simulink model "Pyramidal_Config_Model"  (R2024b)
settings: Solver=VariableStepAuto  StartTime=0.0  StopTime=50  FixedStep=0.001  RelTol=1e-3
libraries: slpidlib x7, simulink_extras x2, aerolibutil x1
settings Model: Creator=LEGION  LastModifiedBy=LEGION

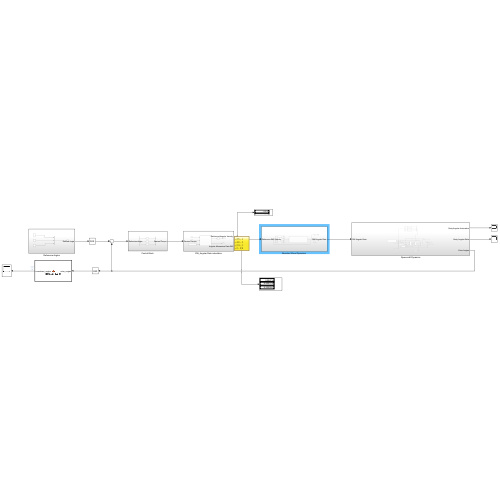
[thumbnail: Simulink's stored preview of the top-level diagram]
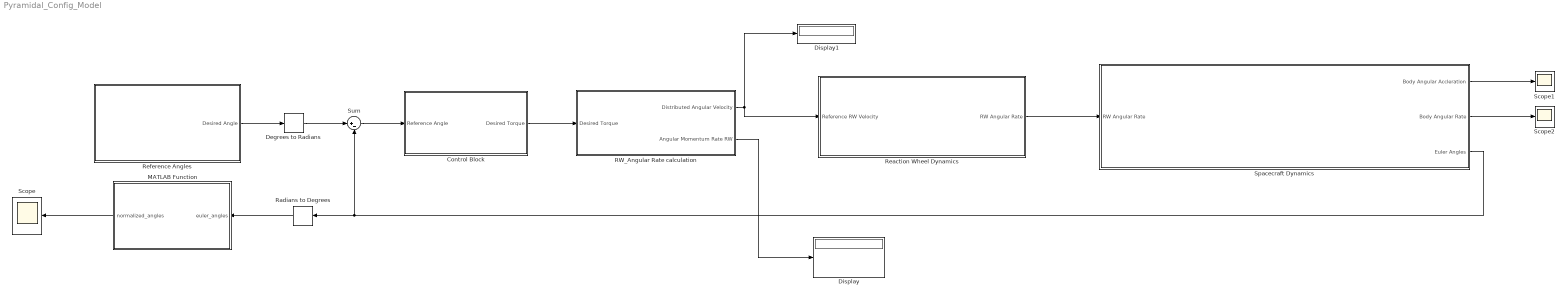
== system Pyramidal_Config_Model ==
  Control Block : Subsystem
  Degrees to Radians : simulink_extras/Transformations/Degrees to Radians
  Display : Display
  Display1 : Display
  MATLAB Function : MATLAB Function  TreatAsAtomicUnit=on
  RW_Angular Rate calculation : Subsystem
  Radians to Degrees : simulink_extras/Transformations/Radians to Degrees
  "Reaction Wheel Dynamics " : Subsystem
  Reference Angles : Subsystem
  Scope : Scope
  Scope1 : Scope
  Scope2 : Scope
  Spacecraft Dynamics : Subsystem
  Sum : Sum  Inputs=|+-
  wires:
  Degrees to Radians/1 -> Sum/1
  Sum/1 -> Control Block/1(Reference Angle)
  Control Block/1(Desired Torque) -> RW_Angular Rate calculation/1(Desired Torque)
  RW_Angular Rate calculation/1(Distributed Angular Velocity) -> Display1/1, "Reaction Wheel Dynamics "/1(Reference RW Velocity)
  MATLAB Function/1(normalized_angles) -> Scope/1
  Spacecraft Dynamics/1(Body Angular Accleration) -> Scope1/1
  Spacecraft Dynamics/2(Body Angular Rate) -> Scope2/1
  RW_Angular Rate calculation/2(Angular Momentum Rate RW) -> Display/1
  Spacecraft Dynamics/3(Euler Angles) -> Sum/2, Radians to Degrees/1
  Radians to Degrees/1 -> MATLAB Function/1(euler_angles)
  Reference Angles/1(Desired Angle) -> Degrees to Radians/1
  "Reaction Wheel Dynamics "/1(RW Angular Rate) -> Spacecraft Dynamics/1(RW Angular Rate)

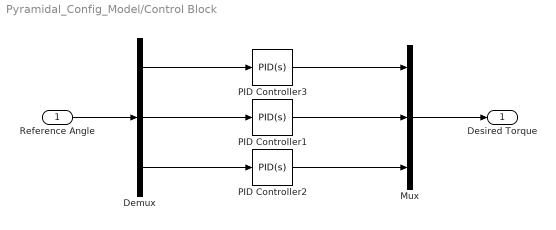
== system Pyramidal_Config_Model/Control Block ==
  Reference Angle : Inport
  Demux : Demux  Outputs=3
  Mux : Mux  Inputs=3
  PID Controller1 : slpidlib/PID Controller  Controller=PID  Form=Parallel  TimeDomain=Continuous-time  UseExternalTs=off  SampleTime=-1  IntegratorMethod=Forward Euler  FilterMethod=Forward Euler  ControllerParametersSource=internal  P=0.1  I=0.05  UseKiTs=off  D=0.01  UseExternalDerivativeSource=off  N=100  UseFilter=on  TunerSelectOption=Transfer Function Based (PID Tuner App)  InitialConditionSource=internal  InitialConditionForIntegrator=0  InitialConditionForFilter=0  DifferentiatorICPrevScaledInput=0  ExternalReset=none  TrackingMode=off  Kt=1  LimitOutput=off  SatLimitsSource=internal  UpperSaturationLimit=inf  LowerSaturationLimit=-inf  LinearizeAsGain=on  AntiWindupMode=none  Kb=1  LimitIntegrator=off  UpperIntegratorSaturationLimit=inf  LowerIntegratorSaturationLimit=-inf  POutMin=[]  POutMax=[]  IOutMin=[]  IOutMax=[]  DOutMin=[]  DOutMax=[]  NOutMin=[]  NOutMax=[]  SumOutMin=[]  SumOutMax=[]  SaturationOutMin=[]  SaturationOutMax=[]  PParamMin=[]  PParamMax=[]  IParamMin=[]  IParamMax=[]  DParamMin=[]  DParamMax=[]  NParamMin=[]  NParamMax=[]  KbParamMin=[]  KbParamMax=[]  KtParamMin=[]  KtParamMax=[]  KbOutMin=[]  KbOutMax=[]  KtOutMin=[]  KtOutMax=[]  IntegratorOutMin=[]  IntegratorOutMax=[]  FilterOutMin=[]  FilterOutMax=[]  SumI1OutMin=[]  SumI1OutMax=[]  SumI2OutMin=[]  SumI2OutMax=[]  SumI3OutMin=[]  SumI3OutMax=[]  SumI4OutMin=[]  SumI4OutMax=[]  SumDOutMin=[]  SumDOutMax=[]  DifferentiatorOutMin=[]  DifferentiatorOutMax=[]  FilterDiffOutCoefMin=[]  FilterDiffOutCoefMax=[]  ReciprocalOutMin=[]  ReciprocalOutMax=[]  SumDenOutMin=[]  SumDenOutMax=[]  SumNumOutMin=[]  SumNumOutMax=[]  DivideOutMin=[]  DivideOutMax=[]  UdiffTsProdOutMin=[]  UdiffTsProdOutMax=[]  NTsProdOutMin=[]  NTsProdOutMax=[]  UintegralTsProdOutMin=[]  UintegralTsProdOutMax=[]  UngainTsProdOutMin=[]  UngainTsProdOutMax=[]  ClampingZeroOutDataTypeStr=Inherit: Inherit via back propagation  ClampingZeroOutMin=[]  ClampingZeroOutMax=[]  FilterDenConstantOutDataTypeStr=Inherit: Inherit via back propagation  FilterDenConstantOutMin=[]  FilterDenConstantOutMax=[]  PCopyOutDataTypeStr=Inherit: Inherit via back propagation  PCopyOutMin=[]  PCopyOutMax=[]  NCopyOutDataTypeStr=Inherit: Inherit via back propagation  NCopyOutMin=[]  NCopyOutMax=[]  IntegratorContinuousStateAttributes=''  IntegratorStateMustResolveToSignalObject=off  IntegratorRTWStateStorageClass=Auto  FilterContinuousStateAttributes=''  FilterStateMustResolveToSignalObject=off  FilterRTWStateStorageClass=Auto  ParallelPVariant=InternalParameters  IdealPVariant=Disabled  IVariant=InternalParameters  DVariant=InternalParameters  IntegratorVariant=Continuous  SatVariant=Disabled  AWVariant=Passthrough  PCopyVariant=Disabled  TRVariant=Disabled  FdbkBlocksVariant=Forward  IdealPFdbkVariant=Disabled  SatFdbkVariant=Disabled  DerivativeFilterVariant=ContFilter  NVariant=InternalParameters  NCopyVariant=Disabled  FilterICVariant=InternalICsFilter  IntegratorICVariant=InternalICs  ExternalResetVariant=Disabled  TRSumVariant=Passthrough  SumFdbkVariant=Disabled  SumVariant=Sum_PID  TsampFilterVariant=InternalTs  TsampNgainVariant=Passthrough  TsampIntegralVariant=Disabled_SignalSpec  ExternalSaturationOutDataTypeStr=Inherit: Same as second input  DerivativeSourceVariant=ErrorSignal  PreIntVariant=InternalPreInt
  PID Controller2 : slpidlib/PID Controller  Controller=PID  Form=Parallel  TimeDomain=Continuous-time  UseExternalTs=off  SampleTime=-1  IntegratorMethod=Forward Euler  FilterMethod=Forward Euler  ControllerParametersSource=internal  P=0.1  I=0.005  UseKiTs=off  D=0.01  UseExternalDerivativeSource=off  N=100  UseFilter=on  TunerSelectOption=Transfer Function Based (PID Tuner App)  InitialConditionSource=internal  InitialConditionForIntegrator=0  InitialConditionForFilter=0  DifferentiatorICPrevScaledInput=0  ExternalReset=none  TrackingMode=off  Kt=1  LimitOutput=off  SatLimitsSource=internal  UpperSaturationLimit=inf  LowerSaturationLimit=-inf  LinearizeAsGain=on  AntiWindupMode=none  Kb=1  LimitIntegrator=off  UpperIntegratorSaturationLimit=inf  LowerIntegratorSaturationLimit=-inf  POutMin=[]  POutMax=[]  IOutMin=[]  IOutMax=[]  DOutMin=[]  DOutMax=[]  NOutMin=[]  NOutMax=[]  SumOutMin=[]  SumOutMax=[]  SaturationOutMin=[]  SaturationOutMax=[]  PParamMin=[]  PParamMax=[]  IParamMin=[]  IParamMax=[]  DParamMin=[]  DParamMax=[]  NParamMin=[]  NParamMax=[]  KbParamMin=[]  KbParamMax=[]  KtParamMin=[]  KtParamMax=[]  KbOutMin=[]  KbOutMax=[]  KtOutMin=[]  KtOutMax=[]  IntegratorOutMin=[]  IntegratorOutMax=[]  FilterOutMin=[]  FilterOutMax=[]  SumI1OutMin=[]  SumI1OutMax=[]  SumI2OutMin=[]  SumI2OutMax=[]  SumI3OutMin=[]  SumI3OutMax=[]  SumI4OutMin=[]  SumI4OutMax=[]  SumDOutMin=[]  SumDOutMax=[]  DifferentiatorOutMin=[]  DifferentiatorOutMax=[]  FilterDiffOutCoefMin=[]  FilterDiffOutCoefMax=[]  ReciprocalOutMin=[]  ReciprocalOutMax=[]  SumDenOutMin=[]  SumDenOutMax=[]  SumNumOutMin=[]  SumNumOutMax=[]  DivideOutMin=[]  DivideOutMax=[]  UdiffTsProdOutMin=[]  UdiffTsProdOutMax=[]  NTsProdOutMin=[]  NTsProdOutMax=[]  UintegralTsProdOutMin=[]  UintegralTsProdOutMax=[]  UngainTsProdOutMin=[]  UngainTsProdOutMax=[]  ClampingZeroOutDataTypeStr=Inherit: Inherit via back propagation  ClampingZeroOutMin=[]  ClampingZeroOutMax=[]  FilterDenConstantOutDataTypeStr=Inherit: Inherit via back propagation  FilterDenConstantOutMin=[]  FilterDenConstantOutMax=[]  PCopyOutDataTypeStr=Inherit: Inherit via back propagation  PCopyOutMin=[]  PCopyOutMax=[]  NCopyOutDataTypeStr=Inherit: Inherit via back propagation  NCopyOutMin=[]  NCopyOutMax=[]  IntegratorContinuousStateAttributes=''  IntegratorStateMustResolveToSignalObject=off  IntegratorRTWStateStorageClass=Auto  FilterContinuousStateAttributes=''  FilterStateMustResolveToSignalObject=off  FilterRTWStateStorageClass=Auto  ParallelPVariant=InternalParameters  IdealPVariant=Disabled  IVariant=InternalParameters  DVariant=InternalParameters  IntegratorVariant=Continuous  SatVariant=Disabled  AWVariant=Passthrough  PCopyVariant=Disabled  TRVariant=Disabled  FdbkBlocksVariant=Forward  IdealPFdbkVariant=Disabled  SatFdbkVariant=Disabled  DerivativeFilterVariant=ContFilter  NVariant=InternalParameters  NCopyVariant=Disabled  FilterICVariant=InternalICsFilter  IntegratorICVariant=InternalICs  ExternalResetVariant=Disabled  TRSumVariant=Passthrough  SumFdbkVariant=Disabled  SumVariant=Sum_PID  TsampFilterVariant=InternalTs  TsampNgainVariant=Passthrough  TsampIntegralVariant=Disabled_SignalSpec  ExternalSaturationOutDataTypeStr=Inherit: Same as second input  DerivativeSourceVariant=ErrorSignal  PreIntVariant=InternalPreInt
  PID Controller3 : slpidlib/PID Controller  Controller=PID  Form=Parallel  TimeDomain=Continuous-time  UseExternalTs=off  SampleTime=-1  IntegratorMethod=Forward Euler  FilterMethod=Forward Euler  ControllerParametersSource=internal  P=0.1  I=0.05  UseKiTs=off  D=0.01  UseExternalDerivativeSource=off  N=100  UseFilter=on  TunerSelectOption=Transfer Function Based (PID Tuner App)  InitialConditionSource=internal  InitialConditionForIntegrator=0  InitialConditionForFilter=0  DifferentiatorICPrevScaledInput=0  ExternalReset=none  TrackingMode=off  Kt=1  LimitOutput=off  SatLimitsSource=internal  UpperSaturationLimit=inf  LowerSaturationLimit=-inf  LinearizeAsGain=on  AntiWindupMode=none  Kb=1  LimitIntegrator=off  UpperIntegratorSaturationLimit=inf  LowerIntegratorSaturationLimit=-inf  POutMin=[]  POutMax=[]  IOutMin=[]  IOutMax=[]  DOutMin=[]  DOutMax=[]  NOutMin=[]  NOutMax=[]  SumOutMin=[]  SumOutMax=[]  SaturationOutMin=[]  SaturationOutMax=[]  PParamMin=[]  PParamMax=[]  IParamMin=[]  IParamMax=[]  DParamMin=[]  DParamMax=[]  NParamMin=[]  NParamMax=[]  KbParamMin=[]  KbParamMax=[]  KtParamMin=[]  KtParamMax=[]  KbOutMin=[]  KbOutMax=[]  KtOutMin=[]  KtOutMax=[]  IntegratorOutMin=[]  IntegratorOutMax=[]  FilterOutMin=[]  FilterOutMax=[]  SumI1OutMin=[]  SumI1OutMax=[]  SumI2OutMin=[]  SumI2OutMax=[]  SumI3OutMin=[]  SumI3OutMax=[]  SumI4OutMin=[]  SumI4OutMax=[]  SumDOutMin=[]  SumDOutMax=[]  DifferentiatorOutMin=[]  DifferentiatorOutMax=[]  FilterDiffOutCoefMin=[]  FilterDiffOutCoefMax=[]  ReciprocalOutMin=[]  ReciprocalOutMax=[]  SumDenOutMin=[]  SumDenOutMax=[]  SumNumOutMin=[]  SumNumOutMax=[]  DivideOutMin=[]  DivideOutMax=[]  UdiffTsProdOutMin=[]  UdiffTsProdOutMax=[]  NTsProdOutMin=[]  NTsProdOutMax=[]  UintegralTsProdOutMin=[]  UintegralTsProdOutMax=[]  UngainTsProdOutMin=[]  UngainTsProdOutMax=[]  ClampingZeroOutDataTypeStr=Inherit: Inherit via back propagation  ClampingZeroOutMin=[]  ClampingZeroOutMax=[]  FilterDenConstantOutDataTypeStr=Inherit: Inherit via back propagation  FilterDenConstantOutMin=[]  FilterDenConstantOutMax=[]  PCopyOutDataTypeStr=Inherit: Inherit via back propagation  PCopyOutMin=[]  PCopyOutMax=[]  NCopyOutDataTypeStr=Inherit: Inherit via back propagation  NCopyOutMin=[]  NCopyOutMax=[]  IntegratorContinuousStateAttributes=''  IntegratorStateMustResolveToSignalObject=off  IntegratorRTWStateStorageClass=Auto  FilterContinuousStateAttributes=''  FilterStateMustResolveToSignalObject=off  FilterRTWStateStorageClass=Auto  ParallelPVariant=InternalParameters  IdealPVariant=Disabled  IVariant=InternalParameters  DVariant=InternalParameters  IntegratorVariant=Continuous  SatVariant=Disabled  AWVariant=Passthrough  PCopyVariant=Disabled  TRVariant=Disabled  FdbkBlocksVariant=Forward  IdealPFdbkVariant=Disabled  SatFdbkVariant=Disabled  DerivativeFilterVariant=ContFilter  NVariant=InternalParameters  NCopyVariant=Disabled  FilterICVariant=InternalICsFilter  IntegratorICVariant=InternalICs  ExternalResetVariant=Disabled  TRSumVariant=Passthrough  SumFdbkVariant=Disabled  SumVariant=Sum_PID  TsampFilterVariant=InternalTs  TsampNgainVariant=Passthrough  TsampIntegralVariant=Disabled_SignalSpec  ExternalSaturationOutDataTypeStr=Inherit: Same as second input  DerivativeSourceVariant=ErrorSignal  PreIntVariant=InternalPreInt
  Desired Torque : Outport
  wires:
  Mux/1 -> Desired Torque/1
  Reference Angle/1 -> Demux/1
  Demux/1 -> PID Controller3/1
  PID Controller3/1 -> Mux/1
  PID Controller1/1 -> Mux/2
  Demux/2 -> PID Controller1/1
  Demux/3 -> PID Controller2/1
  PID Controller2/1 -> Mux/3

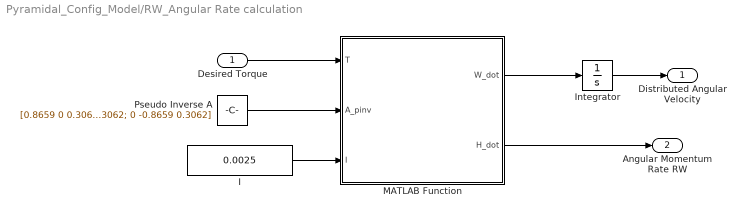
== system Pyramidal_Config_Model/RW_Angular Rate calculation ==
  Desired Torque : Inport
  I : Constant  Value=0.0025  VectorParams1D=off
  Integrator : Integrator
  MATLAB Function : MATLAB Function  TreatAsAtomicUnit=on
  Pseudo Inverse A : Constant  Value=[0.8659 0 0.3062; 0 0.8659 0.3062; -0.8659 0 0.3062; 0 -0.8659 0.3062]  VectorParams1D=off
  Distributed Angular Velocity : Outport
  Angular Momentum Rate RW : Outport  Port=2
  wires:
  MATLAB Function/1(W_dot) -> Integrator/1
  Desired Torque/1 -> MATLAB Function/1(T)
  I/1 -> MATLAB Function/3(I)
  Integrator/1 -> Distributed Angular Velocity/1
  MATLAB Function/2(H_dot) -> Angular Momentum Rate RW/1
  Pseudo Inverse A/1 -> MATLAB Function/2(A_pinv)

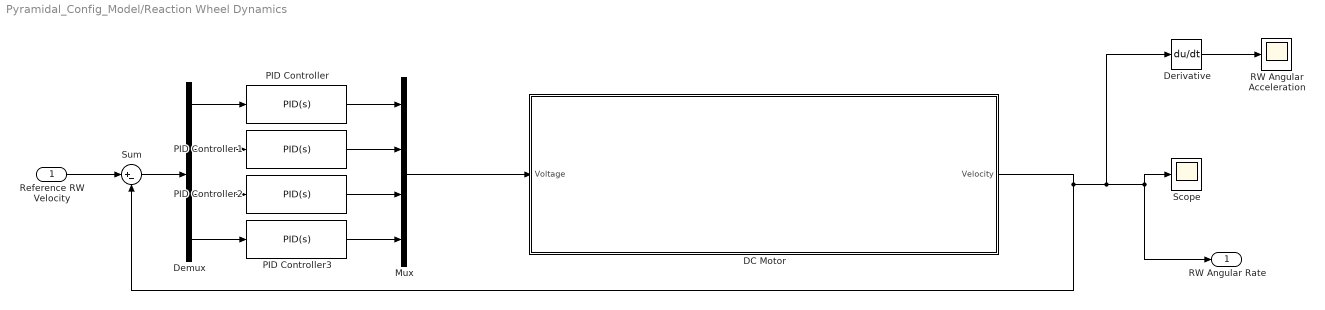
== system Pyramidal_Config_Model/Reaction Wheel Dynamics  ==
  Reference RW Velocity : Inport
  "DC Motor " : Subsystem
  Demux : Demux
  Derivative : Derivative
  Mux : Mux
  PID Controller{,1..3} (4 alike) : slpidlib/PID Controller  Controller=PID  Form=Parallel  TimeDomain=Continuous-time  UseExternalTs=off  SampleTime=-1  IntegratorMethod=Forward Euler  FilterMethod=Forward Euler  ControllerParametersSource=internal  P=0.00016218102087974  I=4.71651669099147e-07  UseKiTs=off  D=0.0223908087939401  UseExternalDerivativeSource=off  N=56.9693255163672  UseFilter=on  TunerSelectOption=Transfer Function Based (PID Tuner App)  InitialConditionSource=internal  InitialConditionForIntegrator=0  InitialConditionForFilter=0  DifferentiatorICPrevScaledInput=0  ExternalReset=none  TrackingMode=off  Kt=1  LimitOutput=off  SatLimitsSource=internal  UpperSaturationLimit=inf  LowerSaturationLimit=-inf  LinearizeAsGain=on  AntiWindupMode=none  Kb=1  LimitIntegrator=off  UpperIntegratorSaturationLimit=inf  LowerIntegratorSaturationLimit=-inf  POutMin=[]  POutMax=[]  IOutMin=[]  IOutMax=[]  DOutMin=[]  DOutMax=[]  NOutMin=[]  NOutMax=[]  SumOutMin=[]  SumOutMax=[]  SaturationOutMin=[]  SaturationOutMax=[]  PParamMin=[]  PParamMax=[]  IParamMin=[]  IParamMax=[]  DParamMin=[]  DParamMax=[]  NParamMin=[]  NParamMax=[]  KbParamMin=[]  KbParamMax=[]  KtParamMin=[]  KtParamMax=[]  KbOutMin=[]  KbOutMax=[]  KtOutMin=[]  KtOutMax=[]  IntegratorOutMin=[]  IntegratorOutMax=[]  FilterOutMin=[]  FilterOutMax=[]  SumI1OutMin=[]  SumI1OutMax=[]  SumI2OutMin=[]  SumI2OutMax=[]  SumI3OutMin=[]  SumI3OutMax=[]  SumI4OutMin=[]  SumI4OutMax=[]  SumDOutMin=[]  SumDOutMax=[]  DifferentiatorOutMin=[]  DifferentiatorOutMax=[]  FilterDiffOutCoefMin=[]  FilterDiffOutCoefMax=[]  ReciprocalOutMin=[]  ReciprocalOutMax=[]  SumDenOutMin=[]  SumDenOutMax=[]  SumNumOutMin=[]  SumNumOutMax=[]  DivideOutMin=[]  DivideOutMax=[]  UdiffTsProdOutMin=[]  UdiffTsProdOutMax=[]  NTsProdOutMin=[]  NTsProdOutMax=[]  UintegralTsProdOutMin=[]  UintegralTsProdOutMax=[]  UngainTsProdOutMin=[]  UngainTsProdOutMax=[]  ClampingZeroOutDataTypeStr=Inherit: Inherit via back propagation  ClampingZeroOutMin=[]  ClampingZeroOutMax=[]  FilterDenConstantOutDataTypeStr=Inherit: Inherit via back propagation  FilterDenConstantOutMin=[]  FilterDenConstantOutMax=[]  PCopyOutDataTypeStr=Inherit: Inherit via back propagation  PCopyOutMin=[]  PCopyOutMax=[]  NCopyOutDataTypeStr=Inherit: Inherit via back propagation  NCopyOutMin=[]  NCopyOutMax=[]  IntegratorContinuousStateAttributes=''  IntegratorStateMustResolveToSignalObject=off  IntegratorRTWStateStorageClass=Auto  FilterContinuousStateAttributes=''  FilterStateMustResolveToSignalObject=off  FilterRTWStateStorageClass=Auto  ParallelPVariant=InternalParameters  IdealPVariant=Disabled  IVariant=InternalParameters  DVariant=InternalParameters  IntegratorVariant=Continuous  SatVariant=Disabled  AWVariant=Passthrough  PCopyVariant=Disabled  TRVariant=Disabled  FdbkBlocksVariant=Forward  IdealPFdbkVariant=Disabled  SatFdbkVariant=Disabled  DerivativeFilterVariant=ContFilter  NVariant=InternalParameters  NCopyVariant=Disabled  FilterICVariant=InternalICsFilter  IntegratorICVariant=InternalICs  ExternalResetVariant=Disabled  TRSumVariant=Passthrough  SumFdbkVariant=Disabled  SumVariant=Sum_PID  TsampFilterVariant=InternalTs  TsampNgainVariant=Passthrough  TsampIntegralVariant=Disabled_SignalSpec  ExternalSaturationOutDataTypeStr=Inherit: Same as second input  DerivativeSourceVariant=ErrorSignal  PreIntVariant=InternalPreInt
  RW Angular Acceleration : Scope
  Scope : Scope
  Sum : Sum  Inputs=|+-
  RW Angular Rate : Outport
  wires:
  Derivative/1 -> RW Angular Acceleration/1
  Reference RW Velocity/1 -> Sum/1
  Sum/1 -> Demux/1
  "DC Motor "/1(Velocity) -> Sum/2, Derivative/1, RW Angular Rate/1, Scope/1
  Mux/1 -> "DC Motor "/1(Voltage)
  PID Controller/1 -> Mux/1
  Demux/1 -> PID Controller/1
  Demux/2 -> PID Controller1/1
  PID Controller1/1 -> Mux/2
  Demux/3 -> PID Controller2/1
  PID Controller2/1 -> Mux/3
  Demux/4 -> PID Controller3/1
  PID Controller3/1 -> Mux/4

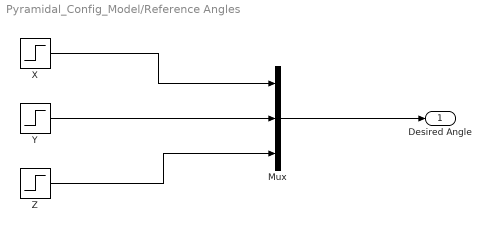
== system Pyramidal_Config_Model/Reference Angles ==
  Mux : Mux  Inputs=3
  X : Step  Time=0.01  After=90  SampleTime=0  VectorParams1D=off
  Y : Step  Time=0.01  After=90  SampleTime=0  VectorParams1D=off
  Z : Step  Time=0.01  After=90  SampleTime=0  VectorParams1D=off
  Desired Angle : Outport
  wires:
  Mux/1 -> Desired Angle/1
  Y/1 -> Mux/2
  Z/1 -> Mux/3
  X/1 -> Mux/1

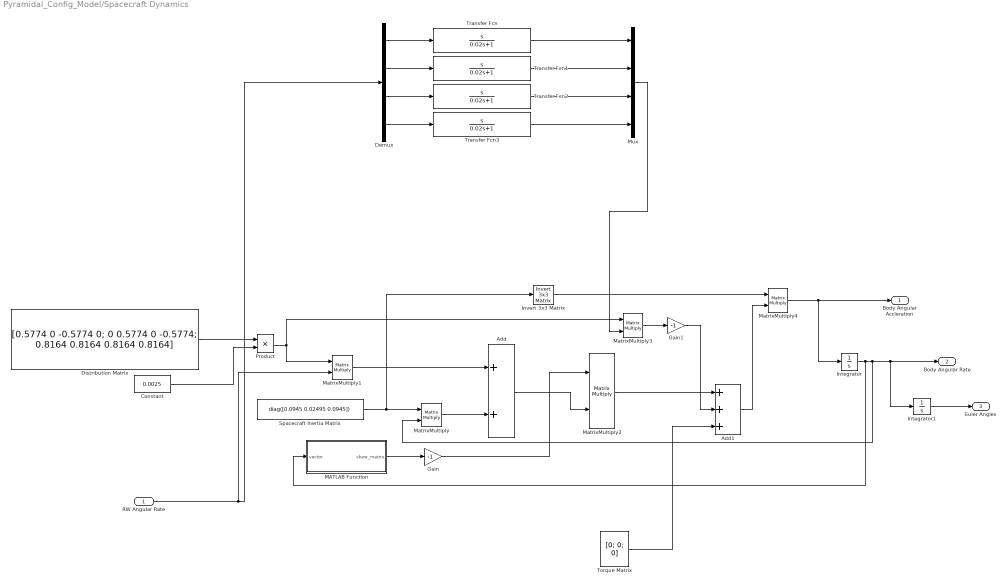
== system Pyramidal_Config_Model/Spacecraft Dynamics ==
  RW Angular Rate : Inport
  Add : Sum
  Add1 : Sum  Inputs=+++
  Constant : Constant  Value=0.0025  VectorParams1D=off
  Demux : Demux
  Distribution Matrix : Constant  Value=[0.5774 0 -0.5774 0; 0 0.5774 0 -0.5774; 0.8164 0.8164 0.8164 0.8164]  VectorParams1D=off
      mask DialogControl Control2 Prompt: (Add text here)
  Gain : Gain  Gain=-1
  Gain1 : Gain  Gain=-1
  Integrator : Integrator
  Integrator1 : Integrator
  Invert 3x3 Matrix : aerolibutil/Invert  3x3 Matrix
  MATLAB Function : MATLAB Function  TreatAsAtomicUnit=on
  MatrixMultiply{,1..4} (5 alike) : Product  Multiplication=Matrix(*)
  Mux : Mux
  Product : Product
  "Spacecraft Inertia Matrix " : Constant  Value=diag([0.0945 0.02495 0.0945])  VectorParams1D=off
  Torque Matrix : Constant  Value=[0; 0; 0]  VectorParams1D=off
  Transfer Fcn{,1..3} (4 alike) : TransferFcn  Numerator=[1 0]  Denominator=[0.02 1]
  Body Angular Accleration : Outport
  Body Angular Rate : Outport  Port=2
  Euler Angles : Outport  Port=3
  wires:
  RW Angular Rate/1 -> Demux/1, MatrixMultiply1/2
  Integrator1/1 -> Euler Angles/1
  MATLAB Function/1(skew_matrix) -> Gain/1
  "Spacecraft Inertia Matrix "/1 -> Invert 3x3 Matrix/1, MatrixMultiply/1
  MatrixMultiply/1 -> Add/2
  Distribution Matrix/1 -> Product/1
  Constant/1 -> Product/2
  Product/1 -> MatrixMultiply3/1, MatrixMultiply1/1
  MatrixMultiply1/1 -> Add/1
  MatrixMultiply2/1 -> Add1/1
  MatrixMultiply3/1 -> Gain1/1
  Gain1/1 -> Add1/2
  Invert 3x3 Matrix/1 -> MatrixMultiply4/1
  Add1/1 -> MatrixMultiply4/2
  MatrixMultiply4/1 -> Integrator/1, Body Angular Accleration/1
  Integrator/1 -> MATLAB Function/1(vector), MatrixMultiply/2, Integrator1/1, Body Angular Rate/1
  Gain/1 -> MatrixMultiply2/1
  Add/1 -> MatrixMultiply2/2
  Demux/1 -> Transfer Fcn/1
  Demux/2 -> Transfer Fcn1/1
  Demux/3 -> Transfer Fcn2/1
  Demux/4 -> Transfer Fcn3/1
  Transfer Fcn3/1 -> Mux/4
  Transfer Fcn2/1 -> Mux/3
  Transfer Fcn1/1 -> Mux/2
  Transfer Fcn/1 -> Mux/1
  Mux/1 -> MatrixMultiply3/2
  Torque Matrix/1 -> Add1/3

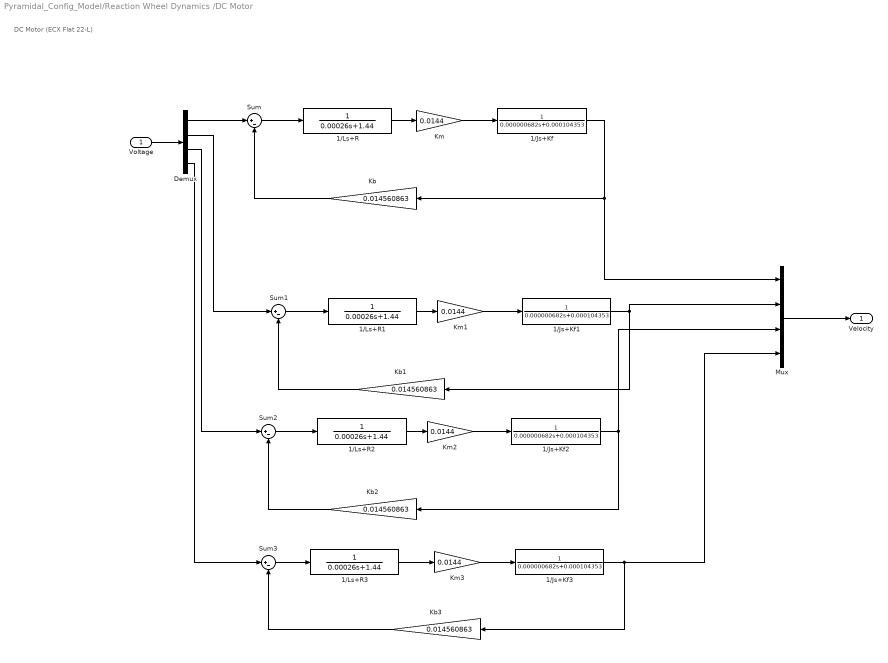
== system Pyramidal_Config_Model/Reaction Wheel Dynamics /DC Motor  ==
  note: DC Motor (ECX Flat 22-L)
  Voltage : Inport
  1/Js+Kf{,1..3} (4 alike) : TransferFcn  Denominator=[0.000000682 0.000104353]
  1/Ls+R{,1..3} (4 alike) : TransferFcn  Denominator=[0.00026 1.44]
  Demux : Demux
  Kb{,1..3} (4 alike) : Gain  Gain=0.014560863
  Km{,1..3} (4 alike) : Gain  Gain=0.0144
  Mux : Mux
  Sum{,1..3} (4 alike) : Sum  Inputs=|+-
  Velocity : Outport
  wires:
  Sum/1 -> 1/Ls+R/1
  1/Ls+R/1 -> Km/1
  Km/1 -> 1/Js+Kf/1
  Kb/1 -> Sum/2
  Voltage/1 -> Demux/1
  Demux/1 -> Sum/1
  Km1/1 -> 1/Js+Kf1/1
  Demux/2 -> Sum1/1
  Kb1/1 -> Sum1/2
  1/Ls+R1/1 -> Km1/1
  1/Js+Kf1/1 -> Kb1/1, Mux/2
  Sum1/1 -> 1/Ls+R1/1
  Km2/1 -> 1/Js+Kf2/1
  Demux/3 -> Sum2/1
  1/Ls+R2/1 -> Km2/1
  1/Js+Kf2/1 -> Kb2/1, Mux/3
  Sum2/1 -> 1/Ls+R2/1
  1/Js+Kf/1 -> Kb/1, Mux/1
  Mux/1 -> Velocity/1
  Kb2/1 -> Sum2/2
  Demux/4 -> Sum3/1
  Sum3/1 -> 1/Ls+R3/1
  1/Ls+R3/1 -> Km3/1
  Km3/1 -> 1/Js+Kf3/1
  1/Js+Kf3/1 -> Kb3/1, Mux/4
  Kb3/1 -> Sum3/2

== matlab function Pyramidal_Config_Model/Spacecraft Dynamics/MATLAB Function ==
  data: vector input; skew_matrix output
function skew_matrix = compute_skew(vector)
    % COMPUTE_SKEW Computes the skew-symmetric matrix of a 3x1 vector.
    %
    % Inputs:
    %   vector - 3x1 input vector
    % Outputs:
    %   skew_matrix - 3x3 skew-symmetric matrix

    % Validate the input dimensions
    if size(vector, 1) ~= 3 || size(vector, 2) ~= 1
        error('Input must be a 3x1 vector.');
    end

    % Extract components of the vector
    x = vector(1);
    y = vector(2);
    z = vector(3);

    % Construct the skew-symmetric matrix
    skew_matrix = [  0, -z,  y;
                     z,  0, -x;
                    -y,  x,  0];
end

== matlab function Pyramidal_Config_Model/RW_Angular Rate calculation/MATLAB Function ==
  data: T input; W_dot output; A_pinv input; I input; H_dot output
function [W_dot, H_dot] = compute_W_dot_and_H_dot(T, A_pinv, I)
    % COMPUTE_W_DOT_AND_H_DOT Computes the angular rate of change of reaction wheels (W_dot)
    % and the rate of change of angular momentum (H_dot) using the precalculated Penrose pseudoinverse.
    %
    % Inputs:
    %   T - 3x1 vector of desired torques (Nm)
    %   A_pinv - 4x3 precalculated Penrose pseudoinverse of the distribution matrix A
    %   I - scalar, moment of inertia of the reaction wheels (kg*m^2)
    %
    % Outputs:
    %   W_dot - 4x1 vector of angular rate of change of the reaction wheels (rad/s^2)
    %   H_dot - 3x1 vector of rate of change of angular momentum (Nm)

    % Validate inputs
    if size(T, 1) ~= 3 || size(A_pinv, 1) ~= 4 || size(A_pinv, 2) ~= 3
        error('Invalid input dimensions. T must be 3x1, and A_pinv must be 4x3.');
    end

    % Compute H_dot (rate of change of angular momentum)
    H_dot = -T;

    % Compute W_dot using the relationship H_dot = A * I * W_dot
    % Rearrange: W_dot = (1/I) * A_pinv * H_dot
    W_dot = (1 / I) * A_pinv * H_dot;

    % Display the results
    disp('The rate of change of angular momentum (H_dot) is:');
    disp(H_dot);
    disp('The angular rate of change of reaction wheels (W_dot) is:');
    disp(W_dot);
end

== matlab function Pyramidal_Config_Model/MATLAB Function ==
  data: euler_angles input; normalized_angles output
function normalized_angles = NormalizedEuler(euler_angles)
% NORMALIZE_EULER_ANGLES Normalizes Euler angles to the range [-180, 180] degrees.
% Input:
%   euler_angles - Nx3 matrix where each row is [x, y, z] Euler angles in degrees
% Output:
%   normalized_angles - Nx3 matrix with normalized Euler angles in the range [-180, 180] degrees

    % Ensure angles are within [-180, 180]
    normalized_angles = mod(euler_angles + 180, 360) - 180;

end
